simulink model "bungee"  (R2023b)
settings: Solver=VariableStepAuto  StartTime=0.0  StopTime=50  MaxStep=0.1  RelTol=1e-3
values from neighbouring files (symbols this model uses):
  a1 = 1.3    [ep6_bungee.m]    (also in ep_6_5_3.m)
  a2 = 1.1    [ep6_bungee.m]    (also in ep_6_5_3.m)
  g = 9.8    [ep6_bungee.m]    (also in ep_6_5_3.m)
  h = 80    [ep6_bungee.m]    (also in ep_6_5_3.m)
  k = 18.45    [ep_6_5_3.m]
  m = 70    [ep6_bungee.m]    (also in ep_6_5_3.m)
  x0 = 30    [ep6_bungee.m]    (also in ep_6_5_2_m.m = [0;0]; ep_6_5_3.m)
settings Model: Creator=86186  LastModifiedBy=86186
settings SolverCC: InitialStep=0.01

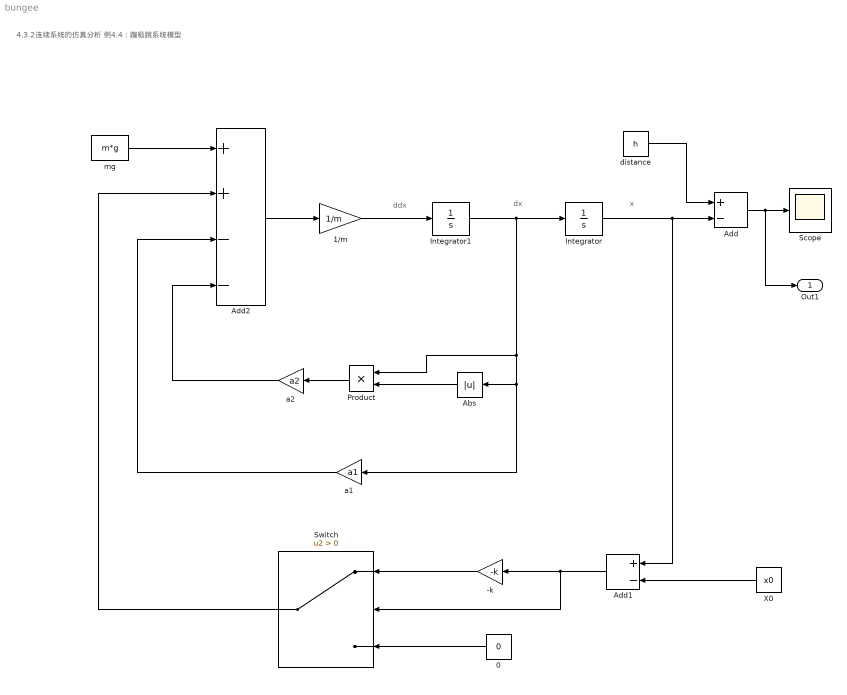
== system bungee ==
  note: dx
  note: ddx
  note: 4.3.2连续系统的仿真分析
      | 例4.4：蹦极跳系统模型
  note: x
  -k : Gain  Gain=-k
  0 : Constant  Value=0
  1/m : Gain  Gain=1/m
  Abs : Abs  SaturateOnIntegerOverflow=off
  Add : Sum  Inputs=+-
  Add1 : Sum  Inputs=+-
  Add2 : Sum  Inputs=++--
  Integrator : Integrator
  Integrator1 : Integrator
  Product : Product
  Scope : Scope
  Switch : Switch  Criteria=u2 > Threshold  SaturateOnIntegerOverflow=off  InputSameDT=off
  X0 : Constant  Value=x0
  a1 : Gain  Gain=a1
  a2 : Gain  Gain=a2
  distance : Constant  Value=h
  mg : Constant  Value=m*g
  Out1 : Outport
  wires:
  Add2/1 -> 1/m/1
  1/m/1 -> Integrator1/1
  Integrator1/1 -> Product/1, a1/1, Abs/1, Integrator/1
  Integrator/1 -> Add1/1, Add/2
  distance/1 -> Add/1
  Add/1 -> Out1/1, Scope/1
  Abs/1 -> Product/2
  Product/1 -> a2/1
  a2/1 -> Add2/4
  a1/1 -> Add2/3
  mg/1 -> Add2/1
  Switch/1 -> Add2/2
  -k/1 -> Switch/1
  Add1/1 -> Switch/2, -k/1
  0/1 -> Switch/3
  X0/1 -> Add1/2
